simulink model "inv_dyn_task_space"  (R2020a)
settings: Solver=VariableStepAuto  StartTime=0.0  StopTime=10.0  RelTol=1e-3
settings Model: Creator=doble  LastModifiedBy=doble

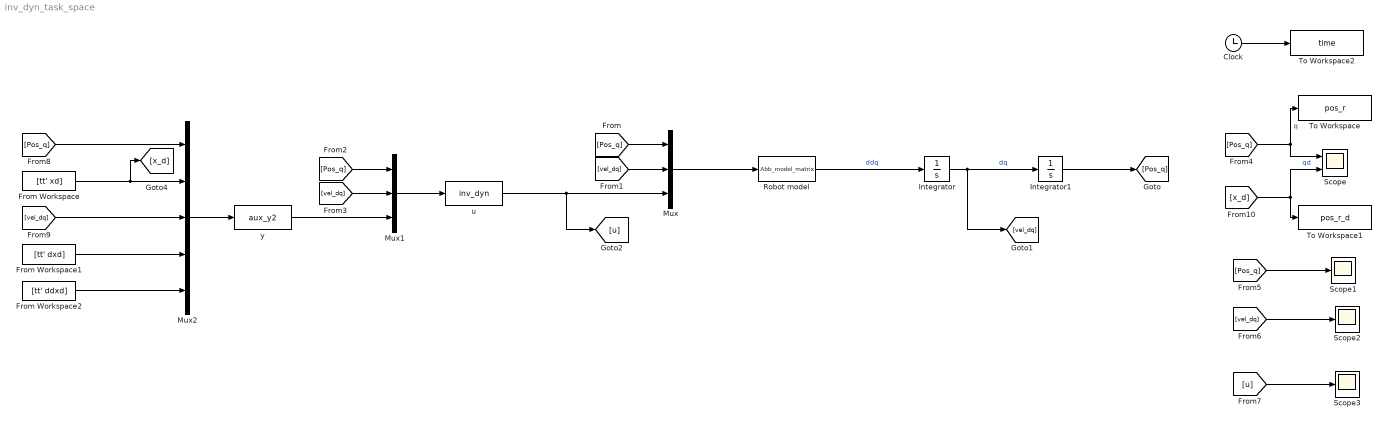
== system inv_dyn_task_space ==
  Clock : Clock
  From Workspace : FromWorkspace  VariableName=[tt' xd]
  From Workspace1 : FromWorkspace  VariableName=[tt' dxd]
  From Workspace2 : FromWorkspace  VariableName=[tt' ddxd]
  Integrator : Integrator
  Integrator1 : Integrator
  Mux : Mux  Inputs=[6 6 6]
  Mux1 : Mux  Inputs=[6 6 6]
  Mux2 : Mux  Inputs=[6 6 6 6 6]
  Robot model : MATLABFcn  MATLABFcn=Abb_model_matrix  OutputDimensions=6
  Scope : Scope  NumInputPorts=2
  Scope1 : Scope
  Scope2 : Scope
  Scope3 : Scope
  To Workspace : ToWorkspace  VariableName=pos_r  SampleTime=-1
  To Workspace1 : ToWorkspace  VariableName=pos_r_d  SampleTime=-1
  To Workspace2 : ToWorkspace  VariableName=time  SampleTime=-1
  "u " : MATLABFcn  MATLABFcn=inv_dyn  OutputDimensions=6
  y : MATLABFcn  MATLABFcn=aux_y2  OutputDimensions=6
  wires:
  Mux/1 -> Robot model/1
  Robot model/1 -> Integrator/1  "ddq"
  Integrator/1 -> [vel_dq], Integrator1/1  "dq"
  Integrator1/1 -> [Pos_q]
  [Pos_q] -> Mux/1
  [vel_dq] -> Mux/2
  "u "/1 -> [u], Mux/3
  Mux1/1 -> "u "/1
  [Pos_q] -> Mux1/1
  [vel_dq] -> Mux1/2
  y/1 -> Mux1/3
  From Workspace2/1 -> Mux2/5
  [Pos_q] -> Mux2/1
  From Workspace1/1 -> Mux2/4
  [vel_dq] -> Mux2/3
  From Workspace/1 -> [x_d], Mux2/2
  Mux2/1 -> y/1
  [u] -> Scope3/1
  [vel_dq] -> Scope2/1
  [x_d] -> To Workspace1/1, Scope/2  "qd"
  [Pos_q] -> To Workspace/1, Scope/1  "q"
  Clock/1 -> To Workspace2/1
  [Pos_q] -> Scope1/1
